simulink model "Simulation_Quarter_Car"  (R2024b)
settings: Solver=VariableStepAuto  StartTime=0.0  StopTime=10  RelTol=1e-3
undefined symbols (not defined in the file): A_num, B_num, C_lqr, C_num, D_lqr, D_num, K, Kalm
libraries: simulink x20
settings Model: Creator=karan  LastModifiedBy=karan

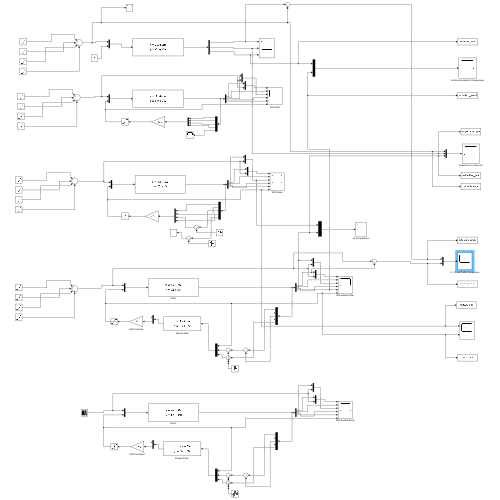
[thumbnail: Simulink's stored preview of the top-level diagram]
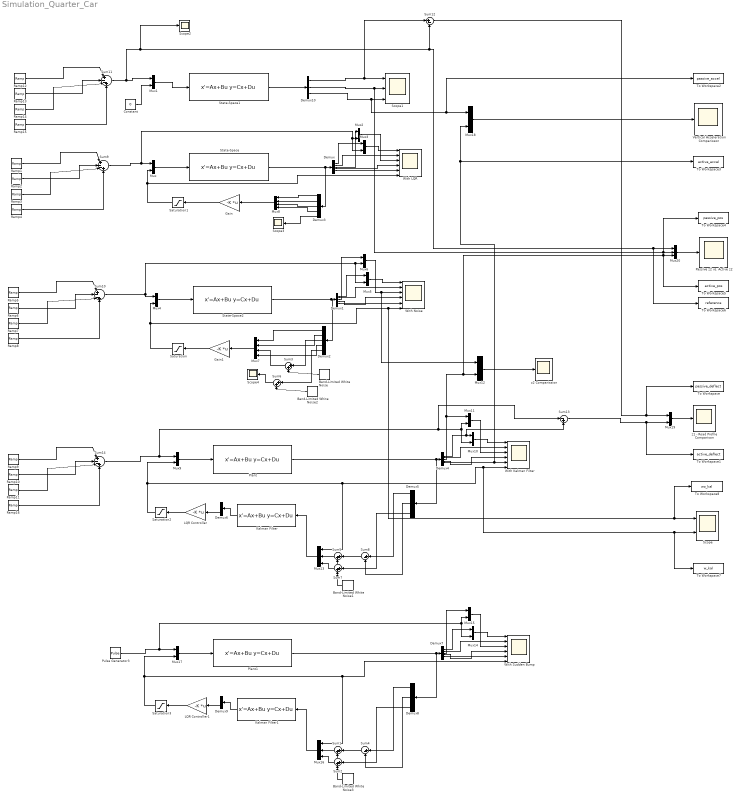
== system Simulation_Quarter_Car ==
  Band-Limited White Noise : simulink/Sources/Band-Limited White Noise  Cov=[0.000001]  Ts=0.001  seed=[23341]
  Band-Limited White Noise1 : simulink/Sources/Band-Limited White Noise  Cov=[0.000001]  Ts=0.1  seed=[23341]
  Band-Limited White Noise2 : simulink/Sources/Band-Limited White Noise  Cov=[0.000001]  Ts=0.001  seed=[23341]
  Band-Limited White Noise3 : simulink/Sources/Band-Limited White Noise  Cov=[0.000001]  Ts=0.1  seed=[23341]
  Constant : Constant  Value=0
  Demux{,1..5,7..8} (8 alike) : Demux  Outputs=5
  Demux10 : Demux  Outputs=3
  Demux6 : Demux  Outputs=[2, 4]
  Demux9 : Demux  Outputs=[2, 4]
  Gain : Gain  Gain=-K  Multiplication=Matrix(K*u)
  Gain1 : Gain  Gain=-K  Multiplication=Matrix(K*u)
  Kalman Filter : StateSpace  A=Kalm.A  B=Kalm.B  C=Kalm.C  D=Kalm.D  InitialCondition=0
  Kalman Filter1 : StateSpace  A=Kalm.A  B=Kalm.B  C=Kalm.C  D=Kalm.D  InitialCondition=0
  LQR Controller : Gain  Gain=-K  Multiplication=Matrix(K*u)
  LQR Controller1 : Gain  Gain=-K  Multiplication=Matrix(K*u)
  Mux{,1..6,9..12,14..15,17..19} (16 alike) : Mux  Inputs=2
  Mux13 : Mux  Inputs=3
  Mux16 : Mux  Inputs=3
  Mux20 : Mux  Inputs=3
  Mux7 : Mux
  Mux8 : Mux
  Passive z2 vs. Active z2 : Scope
  Plant : StateSpace  A=A_num  B=B_num  C=C_lqr  D=D_lqr  InitialCondition=0
  Plant1 : StateSpace  A=A_num  B=B_num  C=C_lqr  D=D_lqr  InitialCondition=0
  Pulse Generator3 : DiscretePulseGenerator  PulseType=Time based  Amplitude=0.02  Period=10  PulseWidth=5  PhaseDelay=1
  Ramp{1,5,9,12} (4 alike) : simulink/Sources/Ramp  slope=0.2667  start=1  InitialOutput=0
  Ramp{2,6,10,13} (4 alike) : simulink/Sources/Ramp  slope=0.2667  start=1.15  InitialOutput=0
  Ramp{3,7,11,14} (4 alike) : simulink/Sources/Ramp  slope=0.2667  start=5.15  InitialOutput=0
  Ramp{4,8,15..16} (4 alike) : simulink/Sources/Ramp  slope=0.2667  start=5.3  InitialOutput=0
  Saturation{,1..3} (4 alike) : Saturate  UpperLimit=3000  LowerLimit=-3000
  Scope : Scope  NumInputPorts=2
  Scope1 : Scope  NumInputPorts=3
  Scope2 : Scope
  Scope3 : Scope
  Scope4 : Scope
  State-Space : StateSpace  A=A_num  B=B_num  C=C_lqr  D=D_lqr  InitialCondition=0
  State-Space1 : StateSpace  A=A_num  B=B_num  C=C_num  D=D_num  InitialCondition=0
  State-Space2 : StateSpace  A=A_num  B=B_num  C=C_lqr  D=D_lqr  InitialCondition=0
  Sum{1..3,5..7} (6 alike) : Sum  Inputs=|++
  Sum{9..11,14} (4 alike) : Sum  Inputs=|+--+
  Sum12 : Sum  Inputs=|+-
  Sum13 : Sum  Inputs=|-+
  Sum4 : Sum  Inputs=|+-
  Sum8 : Sum  Inputs=|+-
  To Workspace : ToWorkspace  VariableName=passive_deflect  SaveFormat=Structure With Time  SampleTime=-1
  To Workspace1 : ToWorkspace  VariableName=active_deflect  SaveFormat=Structure With Time  SampleTime=-1
  To Workspace2 : ToWorkspace  VariableName=passive_accel  SaveFormat=Structure With Time  SampleTime=-1
  To Workspace3 : ToWorkspace  VariableName=active_accel  SaveFormat=Structure With Time  SampleTime=-1
  To Workspace4 : ToWorkspace  VariableName=passive_pos  SaveFormat=Structure With Time  SampleTime=-1
  To Workspace5 : ToWorkspace  VariableName=active_pos  SaveFormat=Structure With Time  SampleTime=-1
  To Workspace6 : ToWorkspace  VariableName=reference  SaveFormat=Structure With Time  SampleTime=-1
  To Workspace7 : ToWorkspace  VariableName=w_kal  SaveFormat=Structure With Time  SampleTime=-1
  To Workspace8 : ToWorkspace  VariableName=wo_kal  SaveFormat=Structure With Time  SampleTime=-1
  Vertical Acceleration Comparisson : Scope
  With Kalman Filter : Scope  NumInputPorts=6
  With LQR : Scope  NumInputPorts=6
  With Noise : Scope  NumInputPorts=6
  With Sudden Bump : Scope  NumInputPorts=6
  z1 - Road Profile Comparison : Scope
  z2 Comparission : Scope
  wires:
  Mux/1 -> State-Space/1
  State-Space/1 -> Demux3/1, Demux/1
  Demux/1 -> Mux3/1
  Demux/2 -> With LQR/2
  Demux/4 -> With LQR/4
  Mux1/1 -> State-Space1/1
  Constant/1 -> Mux1/2
  Sum9/1 -> Mux2/2, Mux3/2, Mux/1
  Demux/3 -> Mux2/1
  Mux2/1 -> With LQR/3
  Mux3/1 -> With LQR/1
  Mux5/1 -> With Noise/1
  Mux6/1 -> Mux12/1, With Noise/3
  Demux1/3 -> Mux6/1
  Sum10/1 -> Mux4/1, Mux5/2, Mux6/2
  Demux1/4 -> With Noise/4
  Demux1/2 -> With Noise/2
  Demux1/1 -> Mux5/1
  State-Space2/1 -> Demux2/1, Demux1/1
  Mux4/1 -> State-Space2/1
  Mux7/1 -> Gain1/1
  Demux2/1 -> Mux7/1
  Demux2/2 -> Mux7/2
  Demux2/4 -> Mux7/4
  Band-Limited White Noise/1 -> Sum3/2
  Demux2/3 -> Sum3/1
  Sum3/1 -> Mux7/3
  Demux/5 -> With LQR/5
  Mux8/1 -> Gain/1
  Demux3/1 -> Mux8/1
  Demux3/2 -> Mux8/2
  Demux3/3 -> Mux8/3
  Demux3/4 -> Mux8/4
  Demux3/5 -> Scope3/1
  Mux9/1 -> Plant/1
  Plant/1 -> Demux4/1, Demux5/1
  Demux4/1 -> Sum13/2, Mux10/1
  Demux4/2 -> With Kalman Filter/2
  Demux4/4 -> With Kalman Filter/4
  Sum14/1 -> Sum13/1, Mux11/2, Mux10/2, Mux9/1
  Demux4/3 -> To Workspace5/1, Mux20/3, Mux12/2, Mux11/1
  Mux11/1 -> With Kalman Filter/3
  Mux10/1 -> With Kalman Filter/1
  Band-Limited White Noise2/1 -> Sum6/2
  Demux2/5 -> Sum6/1
  Sum6/1 -> Scope4/1
  Demux1/5 -> With Noise/5
  Demux4/5 -> Mux18/2, To Workspace3/1, With Kalman Filter/5
  Mux13/1 -> Kalman Filter/1
  Sum7/1 -> Mux13/3
  Sum5/1 -> Mux13/2
  Band-Limited White Noise1/1 -> Sum5/2, Sum7/2
  Demux5/5 -> Sum7/1
  Sum8/1 -> Sum5/1
  Demux5/1 -> Sum8/1
  Demux5/3 -> Sum8/2
  Kalman Filter/1 -> Demux6/1
  Demux6/2 -> LQR Controller/1
  Mux12/1 -> z2 Comparission/1
  Demux9/2 -> LQR Controller1/1
  Kalman Filter1/1 -> Demux9/1
  Demux8/3 -> Sum4/2
  Demux8/1 -> Sum4/1
  Sum4/1 -> Sum1/1
  Demux8/5 -> Sum2/1
  Band-Limited White Noise3/1 -> Sum2/2, Sum1/2
  Sum1/1 -> Mux16/2
  Sum2/1 -> Mux16/3
  Mux16/1 -> Kalman Filter1/1
  Demux7/5 -> With Sudden Bump/5
  Mux14/1 -> With Sudden Bump/1
  Mux15/1 -> With Sudden Bump/3
  Demux7/3 -> Mux15/1
  Pulse Generator3/1 -> Mux17/1, Mux14/2, Mux15/2
  Demux7/4 -> With Sudden Bump/4
  Demux7/2 -> With Sudden Bump/2
  Demux7/1 -> Mux14/1
  Plant1/1 -> Demux8/1, Demux7/1
  Mux17/1 -> Plant1/1
  Gain1/1 -> Saturation/1
  Saturation/1 -> To Workspace8/1, Scope/1, With Noise/6, Mux4/2
  Gain/1 -> Saturation1/1
  Saturation1/1 -> With LQR/6, Mux/2
  LQR Controller/1 -> Saturation2/1
  Saturation2/1 -> Mux9/2, Mux13/1, To Workspace7/1, Scope/2, With Kalman Filter/6
  LQR Controller1/1 -> Saturation3/1
  Saturation3/1 -> Mux16/1, With Sudden Bump/6, Mux17/2
  Ramp15/1 -> Sum11/4
  Ramp14/1 -> Sum11/3
  Ramp12/1 -> Sum11/1
  Ramp13/1 -> Sum11/2
  Sum11/1 -> Scope2/1, To Workspace6/1, Mux20/1, Sum12/2, Mux1/1
  State-Space1/1 -> Demux10/1
  Demux10/1 -> Sum12/1, Scope1/1
  Demux10/2 -> To Workspace4/1, Mux20/2, Scope1/2
  Demux10/3 -> To Workspace2/1, Mux18/1, Scope1/3
  Mux18/1 -> Vertical Acceleration Comparisson/1
  Sum12/1 -> To Workspace/1, Mux19/1
  Sum13/1 -> To Workspace1/1, Mux19/2
  Mux19/1 -> z1 - Road Profile Comparison/1
  Mux20/1 -> Passive z2 vs. Active z2/1
  Ramp2/1 -> Sum9/2
  Ramp1/1 -> Sum9/1
  Ramp3/1 -> Sum9/3
  Ramp4/1 -> Sum9/4
  Ramp8/1 -> Sum10/4
  Ramp7/1 -> Sum10/3
  Ramp5/1 -> Sum10/1
  Ramp6/1 -> Sum10/2
  Ramp10/1 -> Sum14/2
  Ramp9/1 -> Sum14/1
  Ramp11/1 -> Sum14/3
  Ramp16/1 -> Sum14/4
